simulink model "SHE_Bipolar_HB"  (R2023a)
settings: Solver=ode23tb  StartTime=0.0  StopTime=0.02  MaxStep=1e-4  RelTol=1e-3
values from neighbouring files (symbols this model uses):
  t0 = 1e-9    (= 1e-09)    [SHE_Bipolar_HB_Code.m]
  t1 = new_angles(1)*0.02/360    [SHE_Bipolar_HB_Code.m]
  t2 = new_angles(2)*0.02/360    [SHE_Bipolar_HB_Code.m]
libraries: spsSeriesRLCBranchLib x4, spsMosfetLib x2, spsDCVoltageSourceLib x1, simulink x1, spsVoltageMeasurementLib x1, spspowerguiLib x1
settings Model: Creator=gaming3  LastModifiedBy=gaming3

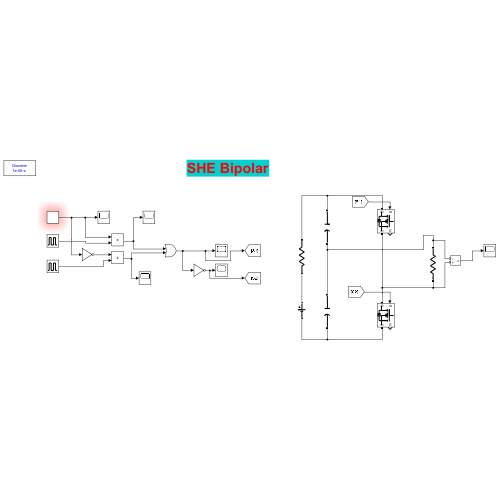
[thumbnail: Simulink's stored preview of the top-level diagram]
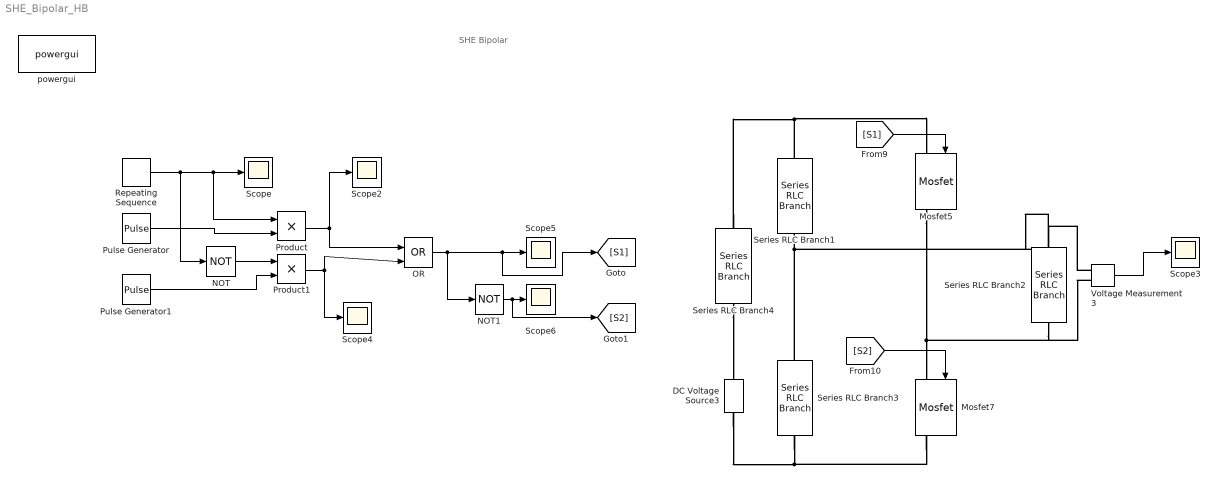
== system SHE_Bipolar_HB ==
  note: SHE Bipolar
  DC Voltage Source3 : spsDCVoltageSourceLib/DC Voltage Source  Amplitude=310  Measurements=None
  Mosfet5 : spsMosfetLib/Mosfet  Ron=0.1  Lon=0  Rd=0.01  Vfd=0  IC=0  Rs=1e5  Cs=inf  Measurements=on
  Mosfet7 : spsMosfetLib/Mosfet  Ron=0.1  Lon=0  Rd=0.01  Vfd=0  IC=0  Rs=1e5  Cs=inf  Measurements=on
  NOT : Logic  Operator=NOT  IconShape=distinctive  AllPortsSameDT=off  OutDataTypeStr=boolean
  NOT1 : Logic  Operator=NOT  IconShape=distinctive  AllPortsSameDT=off  OutDataTypeStr=boolean
  OR : Logic  Operator=OR  IconShape=distinctive  AllPortsSameDT=off  OutDataTypeStr=boolean
  Product : Product
  Product1 : Product
  Pulse Generator : DiscretePulseGenerator  PulseType=Time based  Period=0.02  PulseWidth=50
  Pulse Generator1 : DiscretePulseGenerator  PulseType=Time based  Period=0.02  PulseWidth=50  PhaseDelay=0.01
  Repeating Sequence : simulink/Sources/Repeating Sequence  rep_seq_t=[0 t1 t1+t0 t2 t2+t0 .01/2+t1 .01/2+t1+t0 .01/2+t2 .01/2+t2+t0 .01 ]  rep_seq_y=[1 1 0 0 1 1 0 0 1 1]
  Scope{,2..6} (6 alike) : Scope
  Series RLC Branch1 : spsSeriesRLCBranchLib/Series RLC Branch  LConnTagsString=__new0  RConnTagsString=__new0  BranchType=C  Resistance=100  Inductance=1e-3  SetiL0=off  InitialCurrent=0  Capacitance=1000e-6  Setx0=off  InitialVoltage=0  Measurements=None
  Series RLC Branch2 : spsSeriesRLCBranchLib/Series RLC Branch  LConnTagsString=__new0  RConnTagsString=__new0  BranchType=R  Resistance=100  Inductance=1e-3  SetiL0=off  InitialCurrent=0  Capacitance=1e-6  Setx0=off  InitialVoltage=0  Measurements=None
  Series RLC Branch3 : spsSeriesRLCBranchLib/Series RLC Branch  LConnTagsString=__new0  RConnTagsString=__new0  BranchType=C  Resistance=100  Inductance=1e-3  SetiL0=off  InitialCurrent=0  Capacitance=1000e-6  Setx0=off  InitialVoltage=0  Measurements=None
  Series RLC Branch4 : spsSeriesRLCBranchLib/Series RLC Branch  LConnTagsString=__new0  RConnTagsString=__new0  BranchType=R  Resistance=0.01  Inductance=1e-3  SetiL0=off  InitialCurrent=0  Capacitance=1e-6  Setx0=off  InitialVoltage=0  Measurements=None
  Voltage Measurement3 : spsVoltageMeasurementLib/Voltage Measurement  PhasorSimulation=off  OutputType=Complex  PSBequivalent=0
  powergui : spspowerguiLib/powergui  Priority=1  SimulationMode=Discrete  SampleTime=1e-06  frequency=60  Iterations=50  frequencyindice=0  Pbase=100e6  ErrMax=1e-4  UnitsV=kV  UnitsW=MW  buscounter=0  FunctionMessages=off  echomessages=off  EnableUseOfTLC=off  CurrentSourceSwitches=off  DisableSnubberDevices=off  DisableRonSwitches=off  DisableVfSwitches=off  DisplayEquations=off  AutomaticDiscreteSolvers=off  SolverType=Tustin/Backward Euler (TBE)  Interpol=off  ExternalGateDelay=off  methode=off  Ts=100  x0status=blocks  SPID=on  SwTol=0  HookPort=off  NonlinearTolerance=1e-4  nMaxIteration=100  ContinueOnMaxIteration=off  RestoreLinks=warning  ResistiveCurrentMeasurement=off  Frange=[0:2:500]  Ylog=off  Xlog=on  ShowGrid=off  save=off  variable=ZData  structure=0  ZoomFFT=off  StartTime=0.0  cycles=1  DisplayStyle=1  fundamental=60  FreqAxis=off  MaxFrequency=1000  frequencyindicesteady=1  RmsSteady=1  display=off
  wires:
  Repeating Sequence/1 -> NOT/1, Product/1, Scope/1
  Pulse Generator/1 -> Product/2
  Product/1 -> OR/1, Scope2/1
  Product1/1 -> OR/2, Scope4/1
  NOT/1 -> Product1/1
  Pulse Generator1/1 -> Product1/2
  OR/1 -> NOT1/1, [S1], Scope5/1
  NOT1/1 -> [S2], Scope6/1
  [S1] -> Mosfet5/1
  [S2] -> Mosfet7/1
  Voltage Measurement3/1 -> Scope3/1
  connections:
  Series RLC Branch1/LConn1 -- Series RLC Branch4/LConn1 -- Mosfet5/LConn1
  Mosfet5/RConn1 -- Voltage Measurement3/LConn1 -- Series RLC Branch2/LConn1 -- Mosfet7/LConn1
  Mosfet7/RConn1 -- Series RLC Branch3/RConn1 -- DC Voltage Source3/LConn1
  Series RLC Branch3/LConn1 -- Voltage Measurement3/LConn2 -- Series RLC Branch2/RConn1 -- Series RLC Branch1/RConn1
  Series RLC Branch4/RConn1 -- DC Voltage Source3/RConn1
